simulink model "SE3single_NoC"  (R2021a)
settings: Solver=ode4  StartTime=0.0  StopTime=1000  FixedStep=0.02  RelTol=1e-3
values from neighbouring files (symbols this model uses):
  J2 = 1.08263*10^-3    (= 0.00108263)    [Tao_gC.m]
  mu = 3.986*10^14    (= 398600000000000)    [Tao_gC.m]
  Re = 6378140    [Tao_gC.m]    (also in ge_SE3.m = Rd'*R; plotResult.m = Re(2:end,:); plotResult_n.m = Re_n(2:end,:))
undefined symbols (not defined in the file or in its folder): g0, g_10, J, J1, m, m1, omega_0, p_I0, Pos_cons, R0, v_b0, X, xi0, xi_10, xi_tilde0
settings Model: Creator=泽禹  LastModifiedBy=泽禹
settings DebuggingCC: UnderSpecifiedDimensionMsg=warning

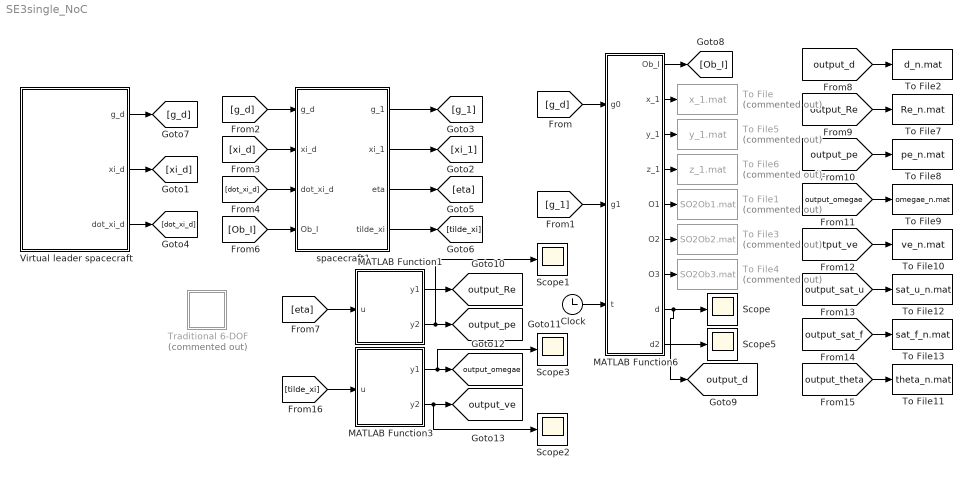
== system SE3single_NoC ==
  Clock : Clock
  MATLAB Function1 : MATLAB Function  TreatAsAtomicUnit=on
  MATLAB Function3 : MATLAB Function  TreatAsAtomicUnit=on
  MATLAB Function6 : MATLAB Function  TreatAsAtomicUnit=on
  Scope{,1..3,5} (5 alike) : Scope
  To File : ToFile  Commented=on  Filename=x_1.mat  MatrixName=x_1
  To File1 : ToFile  Commented=on  Filename=SO2Ob1.mat  MatrixName=SO2Ob1
  To File10 : ToFile  Filename=ve_n.mat  MatrixName=ve_n
  To File11 : ToFile  Filename=theta_n.mat  MatrixName=theta_n
  To File12 : ToFile  Filename=sat_u_n.mat  MatrixName=sat_u_n
  To File13 : ToFile  Filename=sat_f_n.mat  MatrixName=sat_f_n
  To File2 : ToFile  Filename=d_n.mat  MatrixName=d_n
  To File3 : ToFile  Commented=on  Filename=SO2Ob2.mat  MatrixName=SO2Ob2
  To File4 : ToFile  Commented=on  Filename=SO2Ob3.mat  MatrixName=SO2Ob3
  To File5 : ToFile  Commented=on  Filename=y_1.mat  MatrixName=y_1
  To File6 : ToFile  Commented=on  Filename=z_1.mat  MatrixName=z_1
  To File7 : ToFile  Filename=Re_n.mat  MatrixName=Re_n
  To File8 : ToFile  Filename=pe_n.mat  MatrixName=pe_n
  To File9 : ToFile  Filename=omegae_n.mat  MatrixName=omegae_n
  Traditional 6-DOF : Subsystem  Commented=on
  Virtual leader spacecraft : Subsystem
  spacecraft1 : Subsystem
  tag scope: output_Re=global, output_d=global, output_omegae=global, output_pe=global, output_ve=global
  wires:
  Virtual leader spacecraft/1(g_d) -> [g_d]
  Virtual leader spacecraft/2(xi_d) -> [xi_d]
  spacecraft1/1(g_1) -> [g_1]
  spacecraft1/2(xi_1) -> [xi_1]
  [g_d] -> MATLAB Function6/1(g0)
  [g_1] -> MATLAB Function6/2(g1)
  [g_d] -> spacecraft1/1(g_d)
  [xi_d] -> spacecraft1/2(xi_d)
  Virtual leader spacecraft/3(dot_xi_d) -> [dot_xi_d]
  [dot_xi_d] -> spacecraft1/3(dot_xi_d)
  spacecraft1/3(eta) -> [eta]
  spacecraft1/4(tilde_xi) -> [tilde_xi]
  Clock/1 -> MATLAB Function6/3(t)
  MATLAB Function6/1(Ob_I) -> [Ob_I]
  [Ob_I] -> spacecraft1/4(Ob_I)
  MATLAB Function6/2(x_1) -> To File/1
  MATLAB Function6/5(O1) -> To File1/1
  MATLAB Function6/6(O2) -> To File3/1
  MATLAB Function6/7(O3) -> To File4/1
  MATLAB Function6/3(y_1) -> To File5/1
  MATLAB Function6/4(z_1) -> To File6/1
  MATLAB Function6/8(d) -> [output_d], Scope/1
  MATLAB Function3/1(y1) -> Scope3/1, [output_omegae]
  MATLAB Function3/2(y2) -> Scope2/1, [output_ve]
  MATLAB Function1/1(y1) -> [output_Re]
  MATLAB Function1/2(y2) -> Scope1/1, [output_pe]
  MATLAB Function6/9(d2) -> Scope5/1
  [tilde_xi] -> MATLAB Function3/1(u)
  [eta] -> MATLAB Function1/1(u)
  [output_d] -> To File2/1
  [output_Re] -> To File7/1
  [output_pe] -> To File8/1
  [output_omegae] -> To File9/1
  [output_ve] -> To File10/1
  [output_sat_u] -> To File12/1
  [output_sat_f] -> To File13/1
  [output_theta] -> To File11/1

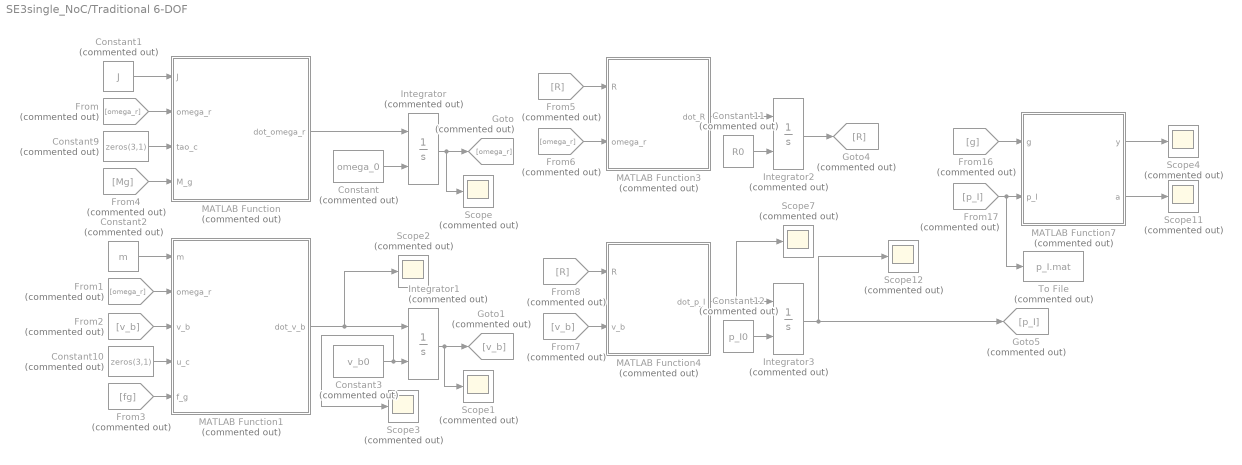
== system SE3single_NoC/Traditional 6-DOF ==
  Constant : Constant  Commented=on  Value=omega_0
  Constant1 : Constant  Commented=on  Value=J
  Constant10 : Constant  Commented=on  Value=zeros(3,1)
  Constant11 : Constant  Commented=on  Value=R0
  Constant12 : Constant  Commented=on  Value=p_I0
  Constant2 : Constant  Commented=on  Value=m
  Constant3 : Constant  Commented=on  Value=v_b0
  Constant9 : Constant  Commented=on  Value=zeros(3,1)
  From : From  Commented=on  GotoTag=omega_r
  From1 : From  Commented=on  GotoTag=omega_r
  From16 : From  Commented=on  GotoTag=g
  From17 : From  Commented=on  GotoTag=p_I
  From2 : From  Commented=on  GotoTag=v_b
  From3 : From  Commented=on  GotoTag=fg
  From4 : From  Commented=on  GotoTag=Mg
  From5 : From  Commented=on  GotoTag=R
  From6 : From  Commented=on  GotoTag=omega_r
  From7 : From  Commented=on  GotoTag=v_b
  From8 : From  Commented=on  GotoTag=R
  Goto : Goto  Commented=on  GotoTag=omega_r
  Goto1 : Goto  Commented=on  GotoTag=v_b
  Goto4 : Goto  Commented=on  GotoTag=R
  Goto5 : Goto  Commented=on  GotoTag=p_I
  Integrator{,1..3} (4 alike) : Integrator  Commented=on  InitialConditionSource=external
  MATLAB Function : MATLAB Function  Commented=on  TreatAsAtomicUnit=on
  MATLAB Function1 : MATLAB Function  Commented=on  TreatAsAtomicUnit=on
  MATLAB Function3 : MATLAB Function  Commented=on  TreatAsAtomicUnit=on
  MATLAB Function4 : MATLAB Function  Commented=on  TreatAsAtomicUnit=on
  MATLAB Function7 : MATLAB Function  Commented=on  TreatAsAtomicUnit=on
  Scope{,1..4,7,11..12} (8 alike) : Scope  Commented=on
  To File : ToFile  Commented=on  Filename=p_I.mat  MatrixName=p_I
  wires:
  Constant/1 -> Integrator/2
  Constant1/1 -> MATLAB Function/1(J)
  From3/1 -> MATLAB Function1/5(f_g)
  Constant2/1 -> MATLAB Function1/1(m)
  Integrator3/1 -> Scope12/1, Goto5/1
  From6/1 -> MATLAB Function3/2(omega_r)
  From17/1 -> To File/1, MATLAB Function7/2(p_I)
  MATLAB Function4/1(dot_p_I) -> Scope7/1, Integrator3/1
  From4/1 -> MATLAB Function/4(M_g)
  Integrator/1 -> Scope/1, Goto/1
  Constant3/1 -> Scope3/1, Integrator1/2
  Constant12/1 -> Integrator3/2
  Constant11/1 -> Integrator2/2
  From/1 -> MATLAB Function/2(omega_r)
  MATLAB Function7/1(y) -> Scope4/1
  Constant9/1 -> MATLAB Function/3(tao_c)
  From1/1 -> MATLAB Function1/2(omega_r)
  From5/1 -> MATLAB Function3/1(R)
  MATLAB Function1/1(dot_v_b) -> Scope2/1, Integrator1/1
  From2/1 -> MATLAB Function1/3(v_b)
  Constant10/1 -> MATLAB Function1/4(u_c)
  MATLAB Function/1(dot_omega_r) -> Integrator/1
  From16/1 -> MATLAB Function7/1(g)
  Integrator1/1 -> Scope1/1, Goto1/1
  MATLAB Function3/1(dot_R) -> Integrator2/1
  Integrator2/1 -> Goto4/1
  From7/1 -> MATLAB Function4/2(v_b)
  From8/1 -> MATLAB Function4/1(R)
  MATLAB Function7/2(a) -> Scope11/1

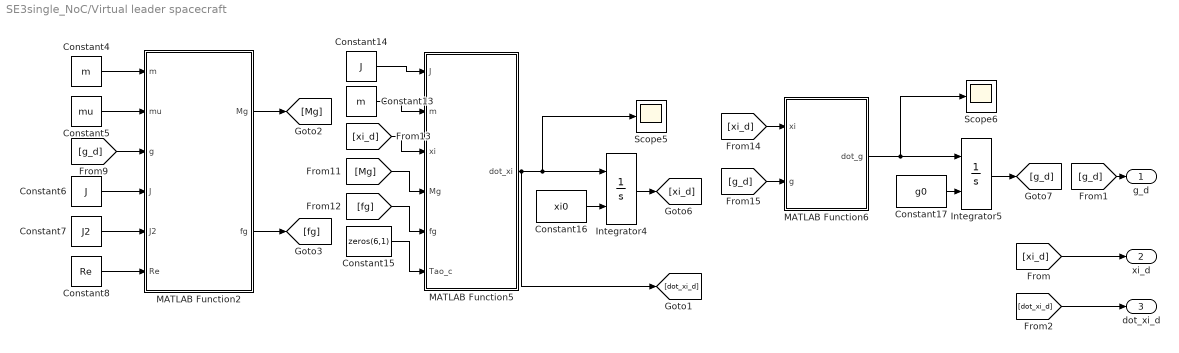
== system SE3single_NoC/Virtual leader spacecraft ==
  Constant13 : Constant  Value=m
  Constant14 : Constant  Value=J
  Constant15 : Constant  Value=zeros(6,1)
  Constant16 : Constant  Value=xi0
  Constant17 : Constant  Value=g0
  Constant4 : Constant  Value=m
  Constant5 : Constant  Value=mu
  Constant6 : Constant  Value=J
  Constant7 : Constant  Value=J2
  Constant8 : Constant  Value=Re
  Integrator4 : Integrator  InitialConditionSource=external
  Integrator5 : Integrator  InitialConditionSource=external
  MATLAB Function2 : MATLAB Function  TreatAsAtomicUnit=on
  MATLAB Function5 : MATLAB Function  TreatAsAtomicUnit=on
  MATLAB Function6 : MATLAB Function  TreatAsAtomicUnit=on
  Scope5 : Scope
  Scope6 : Scope
  g_d : Outport
  xi_d : Outport  Port=2
  dot_xi_d : Outport  Port=3
  wires:
  [Mg] -> MATLAB Function5/4(Mg)
  MATLAB Function5/1(dot_xi) -> [dot_xi_d], Scope5/1, Integrator4/1
  Constant4/1 -> MATLAB Function2/1(m)
  Constant5/1 -> MATLAB Function2/2(mu)
  Constant14/1 -> MATLAB Function5/1(J)
  Constant16/1 -> Integrator4/2
  Constant15/1 -> MATLAB Function5/6(Tao_c)
  [xi_d] -> MATLAB Function5/3(xi)
  MATLAB Function6/1(dot_g) -> Scope6/1, Integrator5/1
  [xi_d] -> MATLAB Function6/1(xi)
  Constant6/1 -> MATLAB Function2/4(J)
  Constant13/1 -> MATLAB Function5/2(m)
  Constant8/1 -> MATLAB Function2/6(Re)
  Constant17/1 -> Integrator5/2
  [g_d] -> MATLAB Function6/2(g)
  MATLAB Function2/2(fg) -> [fg]
  MATLAB Function2/1(Mg) -> [Mg]
  Constant7/1 -> MATLAB Function2/5(J2)
  [fg] -> MATLAB Function5/5(fg)
  Integrator4/1 -> [xi_d]
  [g_d] -> MATLAB Function2/3(g)
  [xi_d] -> xi_d/1
  Integrator5/1 -> [g_d]
  [g_d] -> g_d/1
  [dot_xi_d] -> dot_xi_d/1

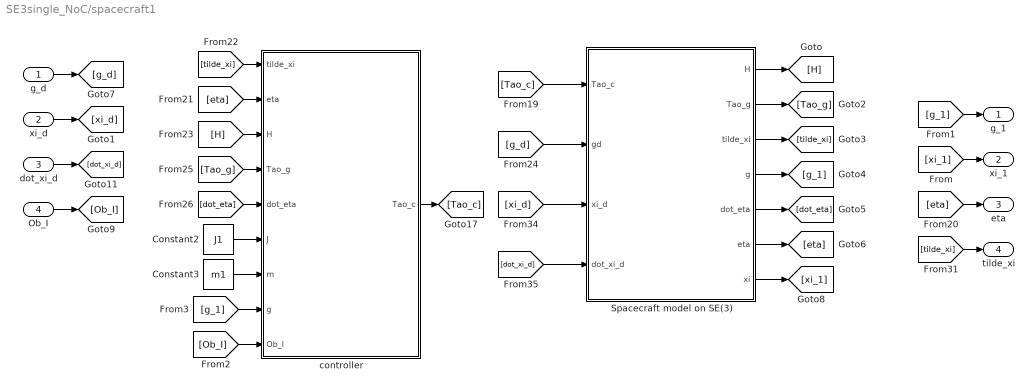
== system SE3single_NoC/spacecraft1 ==
  g_d : Inport
  xi_d : Inport  Port=2
  dot_xi_d : Inport  Port=3
  Ob_I : Inport  Port=4
  Constant2 : Constant  Value=J1
  Constant3 : Constant  Value=m1
  Spacecraft model on SE(3) : Subsystem
  controller : Subsystem
  g_1 : Outport
  xi_1 : Outport  Port=2
  eta : Outport  Port=3
  tilde_xi : Outport  Port=4
  wires:
  g_d/1 -> [g_d]
  xi_d/1 -> [xi_d]
  [xi_1] -> xi_1/1
  [g_1] -> g_1/1
  dot_xi_d/1 -> [dot_xi_d]
  [eta] -> eta/1
  [tilde_xi] -> tilde_xi/1
  [Tao_c] -> Spacecraft model on SE(3)/1(Tao_c)
  [g_d] -> Spacecraft model on SE(3)/2(gd)
  [xi_d] -> Spacecraft model on SE(3)/3(xi_d)
  [dot_xi_d] -> Spacecraft model on SE(3)/4(dot_xi_d)
  Spacecraft model on SE(3)/1(H) -> [H]
  Spacecraft model on SE(3)/2(Tao_g) -> [Tao_g]
  Spacecraft model on SE(3)/3(tilde_xi) -> [tilde_xi]
  Spacecraft model on SE(3)/4(g) -> [g_1]
  Spacecraft model on SE(3)/5(dot_eta) -> [dot_eta]
  Spacecraft model on SE(3)/6(eta) -> [eta]
  Spacecraft model on SE(3)/7(xi) -> [xi_1]
  [tilde_xi] -> controller/1(tilde_xi)
  [eta] -> controller/2(eta)
  [H] -> controller/3(H)
  [Tao_g] -> controller/4(Tao_g)
  [dot_eta] -> controller/5(dot_eta)
  controller/1(Tao_c) -> [Tao_c]
  Constant2/1 -> controller/6(J)
  Constant3/1 -> controller/7(m)
  Ob_I/1 -> [Ob_I]
  [g_1] -> controller/8(g)
  [Ob_I] -> controller/9(Ob_I)

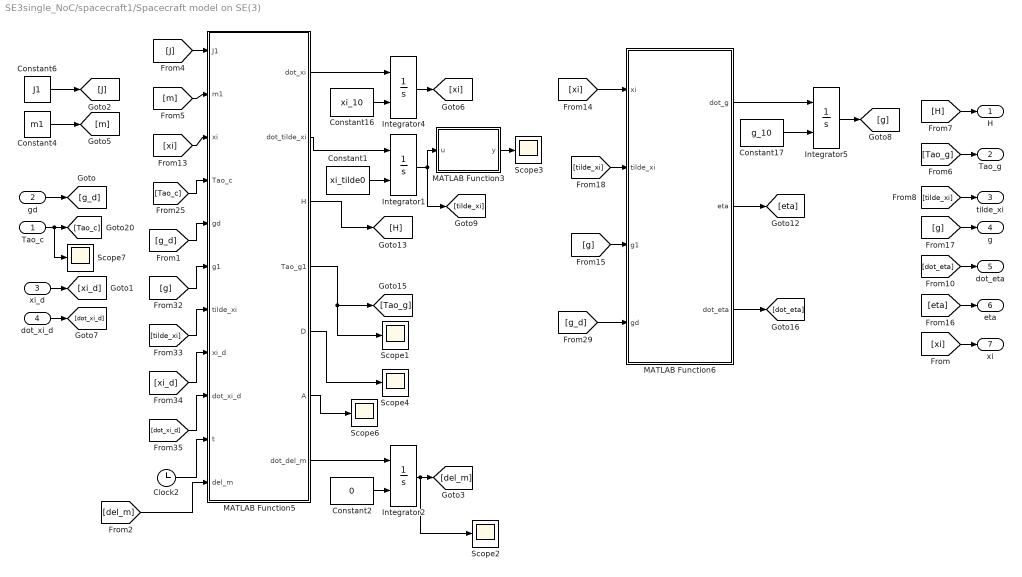
== system SE3single_NoC/spacecraft1/Spacecraft model on SE(3) ==
  Tao_c : Inport
  gd : Inport  Port=2
  xi_d : Inport  Port=3
  dot_xi_d : Inport  Port=4
  Clock2 : Clock
  Constant1 : Constant  Value=xi_tilde0
  Constant16 : Constant  Value=xi_10
  Constant17 : Constant  Value=g_10
  Constant2 : Constant  Value=0
  Constant4 : Constant  Value=m1
  Constant6 : Constant  Value=J1
  Integrator{1..2,4..5} (4 alike) : Integrator  InitialConditionSource=external
  MATLAB Function3 : MATLAB Function  TreatAsAtomicUnit=on
  MATLAB Function5 : MATLAB Function  TreatAsAtomicUnit=on
  MATLAB Function6 : MATLAB Function  TreatAsAtomicUnit=on
  Scope{1..4,6..7} (6 alike) : Scope
  H : Outport
  Tao_g : Outport  Port=2
  tilde_xi : Outport  Port=3
  g : Outport  Port=4
  dot_eta : Outport  Port=5
  eta : Outport  Port=6
  xi : Outport  Port=7
  wires:
  Constant16/1 -> Integrator4/2
  [g] -> MATLAB Function6/3(g1)
  MATLAB Function5/1(dot_xi) -> Integrator4/1
  MATLAB Function5/4(Tao_g1) -> [Tao_g], Scope1/1
  [g_d] -> MATLAB Function6/4(gd)
  MATLAB Function6/1(dot_g) -> Integrator5/1
  [xi] -> MATLAB Function6/1(xi)
  Integrator4/1 -> [xi]
  MATLAB Function5/3(H) -> [H]
  Integrator1/1 -> [tilde_xi], MATLAB Function3/1(u)
  MATLAB Function5/2(dot_tilde_xi) -> Integrator1/1
  Constant6/1 -> [J]
  [Tao_g] -> Tao_g/1
  MATLAB Function6/2(eta) -> [eta]
  Constant4/1 -> [m]
  Constant1/1 -> Integrator1/2
  [g] -> g/1
  [xi] -> MATLAB Function5/3(xi)
  [dot_eta] -> dot_eta/1
  Integrator5/1 -> [g]
  [H] -> H/1
  Constant17/1 -> Integrator5/2
  [g] -> MATLAB Function5/6(g1)
  [tilde_xi] -> MATLAB Function5/7(tilde_xi)
  [tilde_xi] -> MATLAB Function6/2(tilde_xi)
  [tilde_xi] -> tilde_xi/1
  [xi] -> xi/1
  gd/1 -> [g_d]
  [g_d] -> MATLAB Function5/5(gd)
  [xi_d] -> MATLAB Function5/8(xi_d)
  [dot_xi_d] -> MATLAB Function5/9(dot_xi_d)
  xi_d/1 -> [xi_d]
  dot_xi_d/1 -> [dot_xi_d]
  MATLAB Function6/3(dot_eta) -> [dot_eta]
  [J] -> MATLAB Function5/1(J1)
  [m] -> MATLAB Function5/2(m1)
  Tao_c/1 -> Scope7/1, [Tao_c]
  [Tao_c] -> MATLAB Function5/4(Tao_c)
  Clock2/1 -> MATLAB Function5/10(t)
  [eta] -> eta/1
  MATLAB Function3/1(y) -> Scope3/1
  MATLAB Function5/5(D) -> Scope4/1
  MATLAB Function5/6(A) -> Scope6/1
  MATLAB Function5/7(dot_del_m) -> Integrator2/1
  Constant2/1 -> Integrator2/2
  Integrator2/1 -> Scope2/1, [del_m]
  [del_m] -> MATLAB Function5/11(del_m)

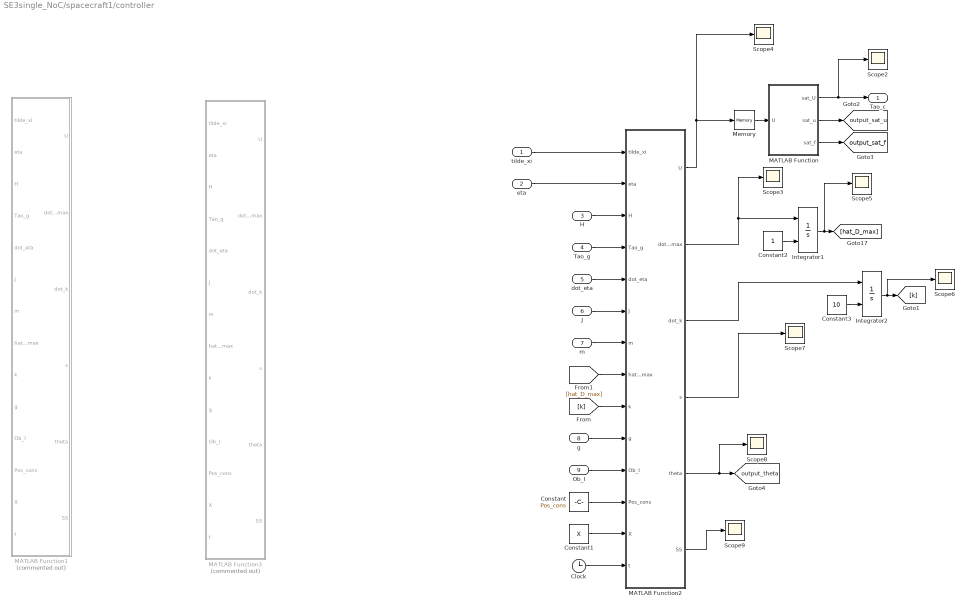
== system SE3single_NoC/spacecraft1/controller ==
  tilde_xi : Inport
  eta : Inport  Port=2
  H : Inport  Port=3
  Tao_g : Inport  Port=4
  dot_eta : Inport  Port=5
  J : Inport  Port=6
  m : Inport  Port=7
  g : Inport  Port=8
  Ob_I : Inport  Port=9
  Clock : Clock
  Constant : Constant  Value=Pos_cons
  Constant1 : Constant  Value=X
  Constant2 : Constant
  Constant3 : Constant  Value=10
  Integrator1 : Integrator  InitialConditionSource=external
  Integrator2 : Integrator  InitialConditionSource=external
  MATLAB Function : MATLAB Function  TreatAsAtomicUnit=on
  MATLAB Function1 : MATLAB Function  Commented=on  TreatAsAtomicUnit=on
  MATLAB Function2 : MATLAB Function  TreatAsAtomicUnit=on
  MATLAB Function3 : MATLAB Function  Commented=on  TreatAsAtomicUnit=on
  Memory : Memory  InitialCondition=zeros(6,1)
  Scope{2..9} (8 alike) : Scope
  Tao_c : Outport
  tag scope: output_sat_f=global, output_sat_u=global, output_theta=global
  wires:
  Tao_g/1 -> MATLAB Function2/4(Tao_g)
  H/1 -> MATLAB Function2/3(H)
  MATLAB Function2/1(U) -> Scope4/1, Memory/1
  m/1 -> MATLAB Function2/7(m)
  tilde_xi/1 -> MATLAB Function2/1(tilde_xi)
  dot_eta/1 -> MATLAB Function2/5(dot_eta)
  J/1 -> MATLAB Function2/6(J)
  Memory/1 -> MATLAB Function/1(U)
  g/1 -> MATLAB Function2/10(g)
  Ob_I/1 -> MATLAB Function2/11(Ob_I)
  Clock/1 -> MATLAB Function2/14(t)
  Constant/1 -> MATLAB Function2/12(Pos_cons)
  Constant1/1 -> MATLAB Function2/13(X)
  MATLAB Function2/2(dot_hat_D_max) -> Integrator1/1, Scope3/1
  MATLAB Function2/3(dot_k) -> Integrator2/1
  Constant2/1 -> Integrator1/2
  Constant3/1 -> Integrator2/2
  Integrator1/1 -> Scope5/1, [hat_D_max]
  Integrator2/1 -> Scope6/1, [k]
  [k] -> MATLAB Function2/9(k)
  [hat_D_max] -> MATLAB Function2/8(hat_D_max)
  MATLAB Function2/4(s) -> Scope7/1
  MATLAB Function/1(sat_U) -> Scope2/1, Tao_c/1
  MATLAB Function2/5(theta) -> [output_theta], Scope8/1
  MATLAB Function2/6(SS) -> Scope9/1
  MATLAB Function/2(sat_u) -> [output_sat_u]
  MATLAB Function/3(sat_f) -> [output_sat_f]
  eta/1 -> MATLAB Function2/2(eta)

== matlab function SE3single_NoC/Virtual leader spacecraft/MATLAB Function6 ==
  data: xi input; dot_g output; g input
function dot_g   = fcn(xi,g)
    dot_g = zeros(4,4);
    
    dot_g = g*x2_hat_se3(xi);

end

== matlab function SE3single_NoC/Traditional 6-DOF/MATLAB Function7 ==
  data: g input; p_I input; y output; a output
function [y,a] = fcn(g,p_I)
%     y = zeros(1,1);
    
    y = g(1:3,4)-p_I;
    a=g(1:3,4);
end

== matlab function SE3single_NoC/MATLAB Function3 ==
  data: u input; y1 output; y2 output
function [y1,y2] = fcn(u)

y1 = norm(rad2deg(u(1:3)));
y2 = norm(u(4:6));

== matlab function SE3single_NoC/spacecraft1/Spacecraft model on SE(3)/MATLAB Function5 ==
  data: dot_xi output; J1 input; m1 input; xi input; Tao_c input; dot_tilde_xi output; gd input; g1 input; tilde_xi input; xi_d input; dot_xi_d input; H output; Tao_g1 output; t input; D output; A output; dot_del_m output; del_m input
function [dot_xi,dot_tilde_xi,H,Tao_g1,D,A,dot_del_m]  = fcn(J1,m1,xi,Tao_c,gd,g1,tilde_xi,xi_d,dot_xi_d,t,del_m)
    dot_xi = zeros(6,1);
    
    d_tao = 10^-2*[1.2+sin(pi/125*t)+sin(pi/200*t);
                  1-sin(pi/125*t)-sin(pi/200*t);
                  1.4+cos(pi/125*t)+cos(pi/200*t)];
    d_f = 10^-3*[4+sin(pi/125*t)+sin(pi/200*t);
                  4.5-sin(pi/125*t)-sin(pi/200*t);
                  3+cos(pi/125*t)+cos(pi/200*t)];
    
    
    Tao_d = [d_tao',d_f']';
    
    
   del_J = zeros(3,3);

   J = zeros(3,3);
   m = zeros(1,1);
   
   del_J = diag([2*sin(0.05*t),2*cos(0.08*t),3*sin(0.02*t)]);

   dot_del_m = 0.0008*norm(Tao_c(4:6));
%    a=norm(Tao_c(4:6));
   
   J = J1+del_J;
   m = m1-del_m;
   
   [Mg,fg] = Tao_gC(m,J,g1);
   [Mg1,fg1] = Tao_gC(m1,J1,g1);
    
   Tao_g = [Mg',fg']';
   Tao_g1 = [Mg1',fg1']';
   
   A= Mg-Mg1;
    
    
    
    
    
    E=zeros(6,6);  % 有不确定性
    E(1:3,1:3)=J;  
    E(4:6,4:6)=m*eye(3);
    
    E1=zeros(6,6);
    E1(1:3,1:3)=J1;  %常量部分
    E1(4:6,4:6)=m1*eye(3);
    
%     [m,n]=eig(inv(E1));
%     max(diag(n));
    
    del_E = inv(E)-inv(E1);

    H1=E\([-x2x_hat(xi(1:3)),zeros(3,3);zeros(3,3),-x2x_hat(xi(1:3))]*E*xi);
%     if t==0
%         dot_xi = E\([-x2x_hat(xi(1:3)),zeros(3,3);zeros(3,3),-x2x_hat(xi(1:3))]*E*xi+Tao_g+Tao_d);
%     else
        dot_xi = E\([-x2x_hat(xi(1:3)),zeros(3,3);zeros(3,3),-x2x_hat(xi(1:3))]*E*xi+Tao_g+Tao_c+Tao_d);
%     end
%     dot_xi2 = E1\([-x2x_hat(xi(1:3)),zeros(3,3);zeros(3,3),-x2x_hat(xi(1:3))]*E1*xi+Tao_g1+Tao_c+Tao_d);
    
%     dot_xi = E\(adstar_xi*E*xi+Tao_g+Tao_c+Tao_d);


    dot_tilde_xi = zeros(6,1); 

    [ge,~,~] = ge_SE3(gd,g1);
    ge_inv =  ge_SE3inv(ge);
    Ad_ge_inv = Adg(ge_inv);
    [adstar_xi,~]=ad(tilde_xi);
    dot_tilde_xi =dot_xi+adstar_xi*Ad_ge_inv*xi_d-Ad_ge_inv*dot_xi_d;
    
    H1=E1\([-x2x_hat(xi(1:3)),zeros(3,3);zeros(3,3),-x2x_hat(xi(1:3))]*E1*xi);
    H2=adstar_xi*Ad_ge_inv*xi_d-Ad_ge_inv*dot_xi_d;
    H=H1+H2;
%     if t==296
%         a=5;
%     end
    D = norm(del_E*([-x2x_hat(xi(1:3)),zeros(3,3);zeros(3,3),-x2x_hat(xi(1:3))]*E*xi+Tao_g+Tao_c)+inv(E1)*([-x2x_hat(xi(1:3)),zeros(3,3);zeros(3,3),-x2x_hat(xi(1:3))]*del_E*xi+Tao_g-Tao_g1)+inv(E)*Tao_d);
end

== matlab function SE3single_NoC/spacecraft1/Spacecraft model on SE(3)/MATLAB Function6 ==
  data: xi input; dot_g output; eta output; tilde_xi input; g1 input; gd input; dot_eta output
function [dot_g,eta,dot_eta]  = fcn(xi,tilde_xi,g1,gd)
    dot_g = zeros(4,4);
    
    dot_g = g1*x2_hat_se3(xi);
    
    dot_eta = zeros(6,1);
    G_eta = zeros(6,6);
 
    [~,Theta_r,eta] = ge_SE3(gd,g1);
%     Theta_r = norm(eta(1:3));
    Phi = eta(1:3);
    Psi = eta(4:6);
    if Theta_r ==0
        A_Phi = eye(3);
        T_Psi = 0.5*x2x_hat(Psi);
        G_eta = [A_Phi,zeros(3,3);T_Psi,A_Phi];
    else
        if abs(Theta_r) == pi
            Theta_r = Theta_r-sign(Theta_r)*0.001;
        end
        A_Phi = eye(3)+0.5*x2x_hat(Phi)+(1/Theta_r^2-(1+cos(Theta_r))/(2*Theta_r*sin(Theta_r)))*(x2x_hat(Phi))^2;
        S_Phi = eye(3)+(1-cos(Theta_r))/Theta_r^2*x2x_hat(Phi)+(Theta_r-sin(Theta_r))/Theta_r^3*x2x_hat(Phi)^2;
        T_Psi = 0.5*x2x_hat(S_Phi*Psi)+(1/Theta_r^2-(1+cos(Theta_r))/(2*Theta_r*sin(Theta_r)))*(Phi*Psi'+Phi'*Psi*A_Phi)...
                -(1+cos(Theta_r))*(Theta_r-sin(Theta_r))/(2*Theta_r*sin(Theta_r)^2)*S_Phi*Psi*Phi'...
                +((1+cos(Theta_r))*(Theta_r+sin(Theta_r))/(2*Theta_r^3*sin(Theta_r)^2)-2/Theta_r^4)*Phi'*Psi*Phi*Phi';
        G_eta = [A_Phi,zeros(3,3);T_Psi,A_Phi];
    end

    dot_eta = G_eta*tilde_xi;
    
end

== matlab function SE3single_NoC/MATLAB Function6 ==
  data: g0 input; g1 input; Ob_I output; x_1 output; t input; y_1 output; z_1 output; O1 output; O2 output; O3 output; d output; d2 output
function [Ob_I,x_1,y_1,z_1,O1,O2,O3,d,d2]  = fcn(g0,g1,t)

    R0 =  g0(1:3,1:3);
    R1 =  g1(1:3,1:3); 
    p0 = g0(1:3,4);
    p1 = g1(1:3,4);
    
    Ob1 = R0'*p0+[60,-1800,30]';
%     Ob2 = R0'*p0+[-320+30*sin(0.1*t),-677-30*cos(0.1*t),150+30*sin(0.1*t)]';
    Ob2 = R0'*p0+[25+30*sin(0.1*t),-800-30*cos(0.1*t),20+30*sin(0.1*t)]';
    
%     Ob3 = R0'*p0+[400,-550,500]';
    Ob3 = R0'*p0+[-20,-550,600]';
%     Ob1 = R0'*p0+[1039.5,-553,904]';
    Ob_I = zeros(3,3);
    Ob_I(:,1)=R0*Ob1;
    Ob_I(:,2)=R0*Ob2;
    Ob_I(:,3)=R0*Ob3;
%     Ob_I(:,4)=R0*Ob4;
    d=zeros(3,1);
    d(1)=norm(p1-Ob_I(:,1));
    d(2)=norm(p1-Ob_I(:,2));
    d(3)=norm(p1-Ob_I(:,3));
%     d(3)=norm(p1-Ob_I(:,3));
    %% 仿真输出
    X = R0'*R1*eye(3);
    x_1 = X(:,1);
    y_1 = X(:,2);
    z_1 = X(:,3);
    
    O1 = Ob1-R0'*p0;
    O2 = Ob2-R0'*p0;
%     O3 = [400,-550,500]';
    O3 = Ob3-R0'*p0;
%     O= [O1,O2,O3]; 
    d2 = R0'*(p1-p0)-[60,-1800,30]';
end

== matlab function SE3single_NoC/MATLAB Function1 ==
  data: u input; y1 output; y2 output
function [y1,y2] = fcn(u)

y1 = norm((u(1:3)));
y2 = norm((u(4:6)));

== matlab function SE3single_NoC/spacecraft1/controller/MATLAB Function1 ==
  data: tilde_xi input; U output; eta input; H input; Tao_g input; dot_eta input; J input; m input; hat_D_max input; k input; g input; Ob_I input; Pos_cons input; X input; t input; dot_hat_D_max output; dot_k output; s output; theta output; SS output
function [U,dot_hat_D_max,dot_k,s,theta,SS]    = fcn(tilde_xi,eta,H,Tao_g,dot_eta,J,m,hat_D_max,k,g,Ob_I,Pos_cons,X,t)
    U=zeros(6,1);
    E=zeros(6,6);
    E(1:3,1:3)=J;
    E(4:6,4:6)=m*eye(3);
        
    v1=diag([0.1,0.1,0.1,0.01,0.01,0.01]);
    v2=diag([0.001,0.001,0.001,0.001,0.001,0.001]);
%     k1=5*eye(6);
    k1=diag([20,20,20,20,20,20]);
    alpha = 0.8;
    sig_alpha =zeros(6,1);
    eta_alpha1 = zeros(6,6);
    labmda_max_E = 110;
    for i=1:size(eta,1)
       sig_alpha(i)=((abs(eta(i)))^alpha)*sign(eta(i));
       eta_alpha1(i,i)=(abs(eta(i)))^(alpha-1);
    end
    s=tilde_xi+v1*eta+v2*sig_alpha;
    U= -E*(H+v1*dot_eta+alpha*v2*eta_alpha1*dot_eta)-Tao_g-k1*s-(labmda_max_E*hat_D_max*s)/(norm(s)+k^2);
    
    beta = 0.0001;
    dot_hat_D_max = 0;
    ksi = 2.25;
    del_ksi = 0.2;
    if hat_D_max^2<ksi 
        dot_hat_D_max = beta*labmda_max_E*norm(s);
    end
    if hat_D_max^2>=ksi 
        dot_hat_D_max = beta*(labmda_max_E*norm(s)-((hat_D_max^2-ksi)*labmda_max_E*norm(s)*hat_D_max)*hat_D_max/(del_ksi*hat_D_max^2));
    end
    
    k2 = 0.0001;
    dot_k = -(k2*labmda_max_E*k*norm(s))*hat_D_max/(norm(s)+k^2);
    
    sat_k = 0.01;
    u_sat = 1;
    f_sat = 20;
    
    M1 = u_sat/sat_k; %力矩饱和
    M2 = f_sat/sat_k;  %力饱和
    
    L_u_temp =zeros(3,M1);
    for i=1:M1
       L_u_temp(1,i)=2/u_sat*DeadZone(sat_k*i,U(1))*sat_k;
       L_u_temp(2,i)=2/u_sat*DeadZone(sat_k*i,U(2))*sat_k;
       L_u_temp(3,i)=2/u_sat*DeadZone(sat_k*i,U(3))*sat_k;
    end
    L_u = zeros(3,1);
    L_u(1)=sum(L_u_temp(1,:));
    L_u(2)=sum(L_u_temp(2,:));
    L_u(3)=sum(L_u_temp(3,:));

    L_f_temp =zeros(3,M2);
    for i=1:M2
       L_f_temp(1,i)=2/f_sat*DeadZone(sat_k*i,U(4))*sat_k;
       L_f_temp(2,i)=2/f_sat*DeadZone(sat_k*i,U(5))*sat_k;
       L_f_temp(3,i)=2/f_sat*DeadZone(sat_k*i,U(6))*sat_k;
    end
    L_f = zeros(3,1);
    L_f(1)=sum(L_f_temp(1,:));
    L_f(2)=sum(L_f_temp(2,:));
    L_f(3)=sum(L_f_temp(3,:));
    
    L = [L_u',L_f']';

    U = 1/2*(U+L);
    %% 考虑障碍物避障
    b= [0;0;1];  %望远镜安装轴
    
    k3 = 5;
    n = Pos_cons(1);
    fo = zeros(3,1);
    Uo = zeros(3,1);
    ra = Pos_cons(3); %避障作用距离
    ro = Pos_cons(2); %与障碍物最小距离
    P = g(1:3,4);
    R = g(1:3,1:3);
    theta1 = zeros(size(Ob_I,2),1);
    for i=1:size(Ob_I,2)
        Po=Ob_I(:,i);
        ri = norm(P-Po);
        if ri >ra
            Uo = Uo+zeros(3,1);
        end
        if ri<= ra
            Uo = Uo+4*(P-Po)*(ra^2-ro^2)*((ri)^2-ra^2)/((ri)^2-ro^2)^3;
        end
    end
    
    fo = -k3*R'*Uo;
%     
    %% 考虑姿态约束
    
    a= [0;0;1];  %望远镜安装轴
    thata_w = deg2rad(10);
    Uf = zeros(3,1);
    theta1 = zeros(3,1);
    for j=1:size(X,1)
       if a'*R'*X(j,1:3)' <cos(X(j,4)) && cos(X(j,4)+thata_w) <=a'*R'*X(j,1:3)' 
            Uf = Uf+(-2*(a'*R'*X(j,1:3)'-cos(X(j,4)+thata_w))*(cos(X(j,4))-cos(X(j,4)+thata_w)))/(a'*R'*X(j,1:3)'-cos(X(j,4)))^3*X(j,1:3)';
       end
       if cos(X(j,4)+thata_w) >a'*R'*X(j,1:3)'
            Uf = Uf+zeros(3,1);
       end
        theta1(j) =rad2deg(acos(a'*R'*X(j,1:3)'));
    end
    
    Ang_C = deg2rad(20);
    thata_w = deg2rad(15);   %% 预警角度rad2deg(0.5*25.5/(norm([1,1,1]))*(deg2rad(10))^2)
    theta2 =zeros(size(Ob_I,2),1);
    for k=1:size(Ob_I,2)
        Po=Ob_I(:,k);
        B = (Po-P)/(norm(Po-P));
        if a'*R'*B <cos(Ang_C) && cos(Ang_C+thata_w) <=a'*R'*B
            Uf = Uf+(-2*(a'*R'*B-cos(Ang_C+thata_w))*(cos(Ang_C)-cos(Ang_C+thata_w)))/(a'*R'*B-cos(Ang_C))^3*B;
        end
        if cos(Ang_C+thata_w) >a'*R'*B
            Uf = Uf+zeros(3,1);
        end
        theta2(k) = rad2deg(acos(b'*R'*B));
    end
%     theta = zeros(7,1);
    theta = [theta1;theta2];
    
    k4 = 0.5;
    
    uf= -k4*Uf;
    
%     M1 = u_sat/sat_k; %力矩饱和
%     M2 = f_sat/sat_k;  %力饱和
%     
%     L_u2_temp =zeros(3,M1);
%     for i=1:M1
%        L_u2_temp(1,i)=2/u_sat*DeadZone(sat_k*i,uf(1))*sat_k;
%        L_u2_temp(2,i)=2/u_sat*DeadZone(sat_k*i,uf(2))*sat_k;
%        L_u2_temp(3,i)=2/u_sat*DeadZone(sat_k*i,uf(3))*sat_k;
%     end
%     L_u2 = zeros(3,1);
%     L_u2(1)=sum(L_u2_temp(1,:));
%     L_u2(2)=sum(L_u2_temp(2,:));
%     L_u2(3)=sum(L_u2_temp(3,:));
% 
%     L_f2_temp =zeros(3,M2);
%     for i=1:M2
%        L_f2_temp(1,i)=2/f_sat*DeadZone(sat_k*i,fo(1))*sat_k;
%        L_f2_temp(2,i)=2/f_sat*DeadZone(sat_k*i,fo(2))*sat_k;
%        L_f2_temp(3,i)=2/f_sat*DeadZone(sat_k*i,fo(3))*sat_k;
%     end
%     L_f2 = zeros(3,1);
%     L_f2(1)=sum(L_f2_temp(1,:));
%     L_f2(2)=sum(L_f2_temp(2,:));
%     L_f2(3)=sum(L_f2_temp(3,:));
%     
%     L_pf = [L_u2',L_f2']';
    
    sat_uf =fcn2(uf,2.5);  %饱和值是1
    sat_fo =fcn2(fo,35);  %饱和值是20
%  
% 
%     U_temp1 = U(1:3);    
%     U_temp1_sat = fcn2(U_temp1,2);
%     U_temp2 = U(4:6);    
%     U_temp2_sat = fcn2(U_temp2,30);
   
    U = U+[sat_uf;sat_fo];
%     U = U;
%     U = [U_temp1_sat;U_temp2_sat]+[sat_uf;sat_fo];
    SS = 20/110*norm(s)-0.0463*norm([sat_uf;sat_fo]);

end

== matlab function SE3single_NoC/spacecraft1/controller/MATLAB Function2 ==
  data: tilde_xi input; U output; eta input; H input; Tao_g input; dot_eta input; J input; m input; hat_D_max input; k input; g input; Ob_I input; Pos_cons input; X input; t input; dot_hat_D_max output; dot_k output; s output; theta output; SS output
function [U,dot_hat_D_max,dot_k,s,theta,SS]    = fcn(tilde_xi,eta,H,Tao_g,dot_eta,J,m,hat_D_max,k,g,Ob_I,Pos_cons,X,t)
    U=zeros(6,1);
    E=zeros(6,6);
    E(1:3,1:3)=J;
    E(4:6,4:6)=m*eye(3);
        
    v1=diag([0.01,0.01,0.01,0.008,0.0012,0.008]*10);
    v2=diag([0.0001,0.0001,0.0001,0.001,0.001,0.001]);
%     k1=5*eye(6);
    k1=diag([20,20,20,20,20,20]*10);
    alpha = 0.8;
    sig_alpha =zeros(6,1);
    eta_alpha1 = zeros(6,6);
    labmda_max_E = 110;
    for i=1:size(eta,1)
       sig_alpha(i)=((abs(eta(i)))^alpha)*sign(eta(i));
       eta_alpha1(i,i)=(abs(eta(i)))^(alpha-1);
    end
    s=tilde_xi+v1*eta+v2*sig_alpha;
    U= -E*(H+v1*dot_eta+alpha*v2*eta_alpha1*dot_eta)-Tao_g-k1*s-(labmda_max_E*hat_D_max*s)/(norm(s)+k^2);
    
    beta = 0.001;
    dot_hat_D_max = 0;
    ksi = 100;
    del_ksi = 10;
    if hat_D_max^2<ksi 
        dot_hat_D_max = beta*labmda_max_E*norm(s);
    end
    if hat_D_max^2>=ksi 
        dot_hat_D_max = beta*(labmda_max_E*norm(s)-((hat_D_max^2-ksi)*labmda_max_E*norm(s)*hat_D_max)*hat_D_max/(del_ksi*hat_D_max^2));
    end
    
    k2 = 0.00001;
    dot_k = -(k2*labmda_max_E*k*norm(s))*hat_D_max/(norm(s)+k^2);
    
    sat_k = 0.01;
    u_sat = 1;
    f_sat = 20;
    
    M1 = u_sat/sat_k; %力矩饱和
    M2 = f_sat/sat_k;  %力饱和
    
    L_u_temp =zeros(3,M1);
    for i=1:M1
       L_u_temp(1,i)=2/u_sat*DeadZone(sat_k*i,U(1))*sat_k;
       L_u_temp(2,i)=2/u_sat*DeadZone(sat_k*i,U(2))*sat_k;
       L_u_temp(3,i)=2/u_sat*DeadZone(sat_k*i,U(3))*sat_k;
    end
    L_u = zeros(3,1);
    L_u(1)=sum(L_u_temp(1,:));
    L_u(2)=sum(L_u_temp(2,:));
    L_u(3)=sum(L_u_temp(3,:));

    L_f_temp =zeros(3,M2);
    for i=1:M2
       L_f_temp(1,i)=2/f_sat*DeadZone(sat_k*i,U(4))*sat_k;
       L_f_temp(2,i)=2/f_sat*DeadZone(sat_k*i,U(5))*sat_k;
       L_f_temp(3,i)=2/f_sat*DeadZone(sat_k*i,U(6))*sat_k;
    end
    L_f = zeros(3,1);
    L_f(1)=sum(L_f_temp(1,:));
    L_f(2)=sum(L_f_temp(2,:));
    L_f(3)=sum(L_f_temp(3,:));
    
    L = [L_u',L_f']';

%     L_u2 = fcn2_L(U(1:3),1);
    
    U = 1/2*(U+L);
    %% 考虑障碍物避障
    b= [0;0;1];  %望远镜安装轴
    
    k3 = 5;
    n = Pos_cons(1);
    fo = zeros(3,1);
    Uo = zeros(3,1);
    ra = Pos_cons(3); %避障作用距离
    ro = Pos_cons(2); %与障碍物最小距离
    P = g(1:3,4);
    R = g(1:3,1:3);
    theta1 = zeros(size(Ob_I,2),1);
    for i=1:size(Ob_I,2)
        Po=Ob_I(:,i);
        ri = norm(P-Po);
        if ri >ra
            Uo = Uo+zeros(3,1);
        end
        if ri<= ra
            Uo = Uo+4*(P-Po)*(ra^2-ro^2)*((ri)^2-ra^2)/((ri)^2-ro^2)^3;
        end
    end
    
    fo = -k3*R'*Uo;
%     
    %% 考虑姿态约束
    
    a= [0;0;1];  %望远镜安装轴
    thata_w = deg2rad(15);
    Uf = zeros(3,1);
    theta1 = zeros(3,1);
    for j=1:size(X,1)
       if a'*R'*X(j,1:3)' <cos(X(j,4)) && cos(X(j,4)+thata_w) <=a'*R'*X(j,1:3)' 
            Uf = Uf+(-2*(a'*R'*X(j,1:3)'-cos(X(j,4)+thata_w))*(cos(X(j,4))-cos(X(j,4)+thata_w)))/(a'*R'*X(j,1:3)'-cos(X(j,4)))^3*X(j,1:3)';
       end
       if cos(X(j,4)+thata_w) >a'*R'*X(j,1:3)'
            Uf = Uf+zeros(3,1);
       end
        theta1(j) =rad2deg(acos(a'*R'*X(j,1:3)'));
    end
    
    Ang_C = deg2rad(15);
    thata_w = deg2rad(15);   %% 预警角度rad2deg(0.5*25.5/(norm([1,1,1]))*(deg2rad(10))^2)
    theta2 =zeros(size(Ob_I,2),1);
    for k=1:size(Ob_I,2)
        Po=Ob_I(:,k);
        B = (Po-P)/(norm(Po-P));
        if a'*R'*B <cos(Ang_C) && cos(Ang_C+thata_w) <=a'*R'*B
            Uf = Uf+(-2*(a'*R'*B-cos(Ang_C+thata_w))*(cos(Ang_C)-cos(Ang_C+thata_w)))/(a'*R'*B-cos(Ang_C))^3*B;
        end
        if cos(Ang_C+thata_w) >a'*R'*B
            Uf = Uf+zeros(3,1);
        end
        theta2(k) = rad2deg(acos(b'*R'*B));
    end
%     theta = zeros(7,1);
    theta = [theta1;theta2];
    
    k4 = 0.001;
    
    uf= -k4*Uf;
    
%     M1 = u_sat/sat_k; %力矩饱和
%     M2 = f_sat/sat_k;  %力饱和
%     
%     L_u2_temp =zeros(3,M1);
%     for i=1:M1
%        L_u2_temp(1,i)=2/u_sat*DeadZone(sat_k*i,uf(1))*sat_k;
%        L_u2_temp(2,i)=2/u_sat*DeadZone(sat_k*i,uf(2))*sat_k;
%        L_u2_temp(3,i)=2/u_sat*DeadZone(sat_k*i,uf(3))*sat_k;
%     end
%     L_u2 = zeros(3,1);
%     L_u2(1)=sum(L_u2_temp(1,:));
%     L_u2(2)=sum(L_u2_temp(2,:));
%     L_u2(3)=sum(L_u2_temp(3,:));
% 
%     L_f2_temp =zeros(3,M2);
%     for i=1:M2
%        L_f2_temp(1,i)=2/f_sat*DeadZone(sat_k*i,fo(1))*sat_k;
%        L_f2_temp(2,i)=2/f_sat*DeadZone(sat_k*i,fo(2))*sat_k;
%        L_f2_temp(3,i)=2/f_sat*DeadZone(sat_k*i,fo(3))*sat_k;
%     end
%     L_f2 = zeros(3,1);
%     L_f2(1)=sum(L_f2_temp(1,:));
%     L_f2(2)=sum(L_f2_temp(2,:));
%     L_f2(3)=sum(L_f2_temp(3,:));
%     
%     L_pf = [L_u2',L_f2']';
    
    sat_uf =fcn2(uf,4);  %饱和值是2
    sat_fo =fcn2(fo,80);  %饱和值是15
%  
% 
    U_temp1 = U(1:3);    
    U_temp1_sat = fcn2(U_temp1,1);
    U_temp2 = U(4:6);    
    U_temp2_sat = fcn2(U_temp2,20);
   
%     U = U+[sat_uf;sat_fo];
    U = U;
%     U = U+1/2*[uf;fo];
%     U = [U_temp1_sat;U_temp2_sat]+1/2*[sat_uf;sat_fo];
    SS = 200/110*norm(s)-0.0463*norm([sat_uf;sat_fo]);

end

== matlab function SE3single_NoC/spacecraft1/controller/MATLAB Function ==
  data: U input; sat_U output; sat_u output; sat_f output
function [sat_U,sat_u,sat_f] = fcn(U)
    sat_U = zeros(6,1);
    sat_U(1:3) =fcn2(U(1:3),1);  %饱和值是1
    sat_U(4:6) =fcn2(U(4:6),20);  %饱和值是20
    
    sat_u = sat_U(1:3);
    sat_f = sat_U(4:6);
end

== matlab function SE3single_NoC/spacecraft1/Spacecraft model on SE(3)/MATLAB Function3 ==
  data: u input; y output
function y = fcn(u)

y = (u(4:6));

== matlab function SE3single_NoC/spacecraft1/controller/MATLAB Function3 ==
  data: tilde_xi input; U output; eta input; H input; Tao_g input; dot_eta input; J input; m input; hat_D_max input; k input; g input; Ob_I input; Pos_cons input; X input; t input; dot_hat_D_max output; dot_k output; s output; theta output; SS output
function [U,dot_hat_D_max,dot_k,s,theta,SS]    = fcn(tilde_xi,eta,H,Tao_g,dot_eta,J,m,hat_D_max,k,g,Ob_I,Pos_cons,X,t)
    U=zeros(6,1);
    E=zeros(6,6);
    E(1:3,1:3)=J;
    E(4:6,4:6)=m*eye(3);
        
    v1=diag([0.01,0.01,0.01,0.008,0.0012,0.008]*10);
    v2=diag([0.0001,0.0001,0.0001,0.001,0.001,0.001]);
%     k1=5*eye(6);
    k1=diag([20,20,20,20,20,20]*10);
    alpha = 0.8;
    sig_alpha =zeros(6,1);
    eta_alpha1 = zeros(6,6);
    labmda_max_E = 110;
    for i=1:size(eta,1)
       sig_alpha(i)=((abs(eta(i)))^alpha)*sign(eta(i));
       eta_alpha1(i,i)=(abs(eta(i)))^(alpha-1);
    end
    s=tilde_xi+v1*eta+v2*sig_alpha;
    U= -E*(H+v1*dot_eta+alpha*v2*eta_alpha1*dot_eta)-Tao_g-k1*s-(labmda_max_E*hat_D_max*s)/(norm(s)+k^2);
    
    beta = 0.01;
    dot_hat_D_max = 0;
    ksi = 900;
    del_ksi = 100;
    if hat_D_max^2<ksi 
        dot_hat_D_max = beta*labmda_max_E*norm(s);
    end
    if hat_D_max^2>=ksi 
        dot_hat_D_max = beta*(labmda_max_E*norm(s)-((hat_D_max^2-ksi)*labmda_max_E*norm(s)*hat_D_max)*hat_D_max/(del_ksi*hat_D_max^2));
    end
    
    k2 = 0.00001;
    dot_k = -(k2*labmda_max_E*k*norm(s))*hat_D_max/(norm(s)+k^2);
    
    sat_k = 0.01;
    u_sat = 1;
    f_sat = 20;
    
    M1 = u_sat/sat_k; %力矩饱和
    M2 = f_sat/sat_k;  %力饱和
    
    L_u_temp =zeros(3,M1);
    for i=1:M1
       L_u_temp(1,i)=2/u_sat*DeadZone(sat_k*i,U(1))*sat_k;
       L_u_temp(2,i)=2/u_sat*DeadZone(sat_k*i,U(2))*sat_k;
       L_u_temp(3,i)=2/u_sat*DeadZone(sat_k*i,U(3))*sat_k;
    end
    L_u = zeros(3,1);
    L_u(1)=sum(L_u_temp(1,:));
    L_u(2)=sum(L_u_temp(2,:));
    L_u(3)=sum(L_u_temp(3,:));

    L_f_temp =zeros(3,M2);
    for i=1:M2
       L_f_temp(1,i)=2/f_sat*DeadZone(sat_k*i,U(4))*sat_k;
       L_f_temp(2,i)=2/f_sat*DeadZone(sat_k*i,U(5))*sat_k;
       L_f_temp(3,i)=2/f_sat*DeadZone(sat_k*i,U(6))*sat_k;
    end
    L_f = zeros(3,1);
    L_f(1)=sum(L_f_temp(1,:));
    L_f(2)=sum(L_f_temp(2,:));
    L_f(3)=sum(L_f_temp(3,:));
    
    L = [L_u',L_f']';

    U = 1/2*(U+L);
    %% 考虑障碍物避障
    b= [0;0;1];  %望远镜安装轴
    
    k3 = 5;
    n = Pos_cons(1);
    fo = zeros(3,1);
    Uo = zeros(3,1);
    ra = Pos_cons(3); %避障作用距离
    ro = Pos_cons(2); %与障碍物最小距离
    P = g(1:3,4);
    R = g(1:3,1:3);
    theta1 = zeros(size(Ob_I,2),1);
    for i=1:size(Ob_I,2)
        Po=Ob_I(:,i);
        ri = norm(P-Po);
        if ri >ra
            Uo = Uo+zeros(3,1);
        end
        if ri<= ra
            Uo = Uo+4*(P-Po)*(ra^2-ro^2)*((ri)^2-ra^2)/((ri)^2-ro^2)^3;
        end
    end
    
    fo = -k3*R'*Uo;
%     
    %% 考虑姿态约束
    
    a= [0;0;1];  %望远镜安装轴
    thata_w = deg2rad(15);
    Uf = zeros(3,1);
    theta1 = zeros(3,1);
    for j=1:size(X,1)
       if a'*R'*X(j,1:3)' <cos(X(j,4)) && cos(X(j,4)+thata_w) <=a'*R'*X(j,1:3)' 
            Uf = Uf+(-2*(a'*R'*X(j,1:3)'-cos(X(j,4)+thata_w))*(cos(X(j,4))-cos(X(j,4)+thata_w)))/(a'*R'*X(j,1:3)'-cos(X(j,4)))^3*X(j,1:3)';
       end
       if cos(X(j,4)+thata_w) >a'*R'*X(j,1:3)'
            Uf = Uf+zeros(3,1);
       end
        theta1(j) =rad2deg(acos(a'*R'*X(j,1:3)'));
    end
    
    Ang_C = deg2rad(15);
    thata_w = deg2rad(15);   %% 预警角度rad2deg(0.5*25.5/(norm([1,1,1]))*(deg2rad(10))^2)
    theta2 =zeros(size(Ob_I,2),1);
    for k=1:size(Ob_I,2)
        Po=Ob_I(:,k);
        B = (Po-P)/(norm(Po-P));
        if a'*R'*B <cos(Ang_C) && cos(Ang_C+thata_w) <=a'*R'*B
            Uf = Uf+(-2*(a'*R'*B-cos(Ang_C+thata_w))*(cos(Ang_C)-cos(Ang_C+thata_w)))/(a'*R'*B-cos(Ang_C))^3*B;
        end
        if cos(Ang_C+thata_w) >a'*R'*B
            Uf = Uf+zeros(3,1);
        end
        theta2(k) = rad2deg(acos(b'*R'*B));
    end
%     theta = zeros(7,1);
    theta = [theta1;theta2];
    
    k4 = 5;
    
    uf= -k4*Uf;
    
%     M1 = u_sat/sat_k; %力矩饱和
%     M2 = f_sat/sat_k;  %力饱和
%     
%     L_u2_temp =zeros(3,M1);
%     for i=1:M1
%        L_u2_temp(1,i)=2/u_sat*DeadZone(sat_k*i,uf(1))*sat_k;
%        L_u2_temp(2,i)=2/u_sat*DeadZone(sat_k*i,uf(2))*sat_k;
%        L_u2_temp(3,i)=2/u_sat*DeadZone(sat_k*i,uf(3))*sat_k;
%     end
%     L_u2 = zeros(3,1);
%     L_u2(1)=sum(L_u2_temp(1,:));
%     L_u2(2)=sum(L_u2_temp(2,:));
%     L_u2(3)=sum(L_u2_temp(3,:));
% 
%     L_f2_temp =zeros(3,M2);
%     for i=1:M2
%        L_f2_temp(1,i)=2/f_sat*DeadZone(sat_k*i,fo(1))*sat_k;
%        L_f2_temp(2,i)=2/f_sat*DeadZone(sat_k*i,fo(2))*sat_k;
%        L_f2_temp(3,i)=2/f_sat*DeadZone(sat_k*i,fo(3))*sat_k;
%     end
%     L_f2 = zeros(3,1);
%     L_f2(1)=sum(L_f2_temp(1,:));
%     L_f2(2)=sum(L_f2_temp(2,:));
%     L_f2(3)=sum(L_f2_temp(3,:));
%     
%     L_pf = [L_u2',L_f2']';
    
    sat_uf =fcn2(uf,4);  %饱和值是2
    sat_fo =fcn2(fo,80);  %饱和值是15
%  
% 
    U_temp1 = U(1:3);    
    U_temp1_sat = fcn2(U_temp1,1);
    U_temp2 = U(4:6);    
    U_temp2_sat = fcn2(U_temp2,20);
   
%     U = U+[sat_uf;sat_fo];
%     U = U;
    U = U+1/2*[uf;fo];
%     U = [U_temp1_sat;U_temp2_sat]+1/2*[sat_uf;sat_fo];
    SS = 200/110*norm(s)-0.0463*norm([sat_uf;sat_fo]);

end

== matlab function SE3single_NoC/Traditional 6-DOF/MATLAB Function1 ==
  data: m input; dot_v_b output; omega_r input; v_b input; u_c input; f_g input
function dot_v_b = fcn(m,omega_r,v_b,u_c,f_g)
    dot_v_b = zeros(3,1);
    d_f = zeros(3,1);
    dot_v_b = (-m*x2x_hat(omega_r)*v_b+u_c+f_g+d_f)/m;
end

== matlab function SE3single_NoC/Traditional 6-DOF/MATLAB Function ==
  data: J input; dot_omega_r output; omega_r input; tao_c input; M_g input
function dot_omega_r = fcn(J,omega_r,tao_c,M_g)
    dot_omega_r = zeros(3,1);
    d_tao = zeros(3,1);
    dot_omega_r = J\(-x2x_hat(omega_r)*J*omega_r+tao_c+M_g+d_tao);
end

== matlab function SE3single_NoC/Virtual leader spacecraft/MATLAB Function2 ==
  data: m input; mu input; Mg output; g input; J input; J2 input; fg output; Re input
function [Mg,fg] = fcn(m,mu,g,J,J2,Re)
    Mg = zeros(3,1);
    fg = zeros(3,1);
    
    R = g(1:3,1:3);
    p = g(1:3,4);
    b = R'*p; 
    
    Mg = 3*(mu/(norm(p))^5)*(x2x_hat(b)*J*b);
    
    J_star = 0.5*trace(J)*eye(3)+J;
    G = -(m*mu/(norm(p))^3)*b-3*(mu/(norm(p))^5)*J_star*b+15/2*(mu*(b'*J*b)/((norm(p))^7))*b;
    f_J2 = m*R'*[-(3*J2*mu*Re^2*p(1))/(2*(norm(p))^5)*(1-5*p(3)/(norm(p))^2);
                 -(3*J2*mu*Re^2*p(2))/(2*(norm(p))^5)*(1-5*p(3)/(norm(p))^2);
                 -(3*J2*mu*Re^2*p(3))/(2*(norm(p))^5)*(3-5*p(3)/(norm(p))^2);];
    fg= G+f_J2;
end

== matlab function SE3single_NoC/Traditional 6-DOF/MATLAB Function3 ==
  data: R input; dot_R output; omega_r input
function dot_R = fcn(R,omega_r)
    dot_R = zeros(3,3);
    dot_R = R*x2x_hat(omega_r);
end

== matlab function SE3single_NoC/Traditional 6-DOF/MATLAB Function4 ==
  data: R input; dot_p_I output; v_b input
function dot_p_I = fcn(R,v_b)
    dot_p_I = zeros(3,1);
    dot_p_I = R*v_b;
end

== matlab function SE3single_NoC/Virtual leader spacecraft/MATLAB Function5 ==
  data: J input; dot_xi output; m input; xi input; Mg input; fg input; Tao_c input
function dot_xi  = fcn(J,m,xi,Mg,fg,Tao_c)
    dot_xi = zeros(6,1);
    
    d_tao = zeros(3,1);
    d_f = zeros(3,1);
    Tao_d = [d_tao',d_f']';
    Tao_g = [Mg',fg']';
    
    E=zeros(6,6);
    E(1:3,1:3)=J;
    E(4:6,4:6)=m*eye(3);
    
    [~,adstar_xi]=ad(xi);
    
   
    bb=adstar_xi*xi;
    

    
    dot_xi = E\([-x2x_hat(xi(1:3)),zeros(3,3);zeros(3,3),-x2x_hat(xi(1:3))]*E*xi+Tao_g+Tao_c+Tao_d);
%     dot_xi = E\(adstar_xi*E*xi+Tao_g+Tao_c+Tao_d);
%     bbb=[-x2x_hat(omega_r)*J*omega_r;-m*x2x_hat(omega_r)*v]-[-x2x_hat(omega_r)*J,zeros(3,3);zeros(3,3),-m*x2x_hat(omega_r)]*[omega_r;v];
%     bbb=adstar_xi*E*xi-[-x2x_hat(omega_r)*J*omega_r;-m*x2x_hat(omega_r)*v];
%    bbb=adstar_xi*E*xi-[-x2x_hat(omega_r)*J,zeros(3,3);zeros(3,3),-m*x2x_hat(omega_r)]*[omega_r;v];
% bbb=-x2x_hat(xi(4:6))*xi(4:6);
end
